simulink model "AEB_Stateflow"  (R2025b)
settings: Solver=ode3  StartTime=0.0  StopTime=15.0  FixedStep=0.001  RelTol=1e-3
values from neighbouring files (symbols this model uses):
  CTRL_DT = 0.01    [AEB_Stateflow_build.m]
  D_BRAKE_L1 = 20.0    (= 20)    [AEB_Stateflow_build.m]
  D_BRAKE_L2 = 10.0    (= 10)    [AEB_Stateflow_build.m]
  D_BRAKE_L3 = 5.0    (= 5)    [AEB_Stateflow_build.m]
  DECEL_BRAKE_L1 = 2.0    (= 2)    [AEB_Stateflow_build.m]
  DECEL_BRAKE_L2 = 4.0    (= 4)    [AEB_Stateflow_build.m]
  DECEL_BRAKE_L3 = 6.0    (= 6)    [AEB_Stateflow_build.m]
  HYSTERESIS_TIME = 0.2    [AEB_Stateflow_build.m]
  POST_BRAKE_TIME = 2.0    (= 2)    [AEB_Stateflow_build.m]
  STEERING_DEG = 5.0    (= 5)    [AEB_Stateflow_build.m]
  TTC_BRAKE_L1 = 3.0    (= 3)    [AEB_Stateflow_build.m]
  TTC_BRAKE_L2 = 2.2    [AEB_Stateflow_build.m]
  TTC_BRAKE_L3 = 1.8    [AEB_Stateflow_build.m]
  TTC_WARNING = 4.0    (= 4)    [AEB_Stateflow_build.m]
  V_EGO_MAX = 16.67    [AEB_Stateflow_build.m]
  V_EGO_MIN = 1.39    [AEB_Stateflow_build.m]
  WARNING_MIN_TIME = 0.8    [AEB_Stateflow_build.m]
settings Model: Creator=rfagu  LastModifiedBy=rfagu

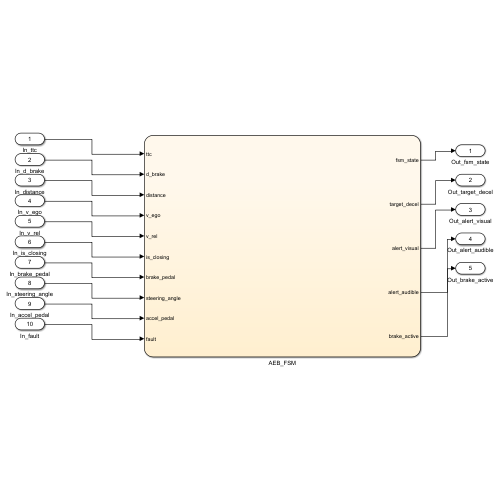
[thumbnail: Simulink's stored preview of the top-level diagram]
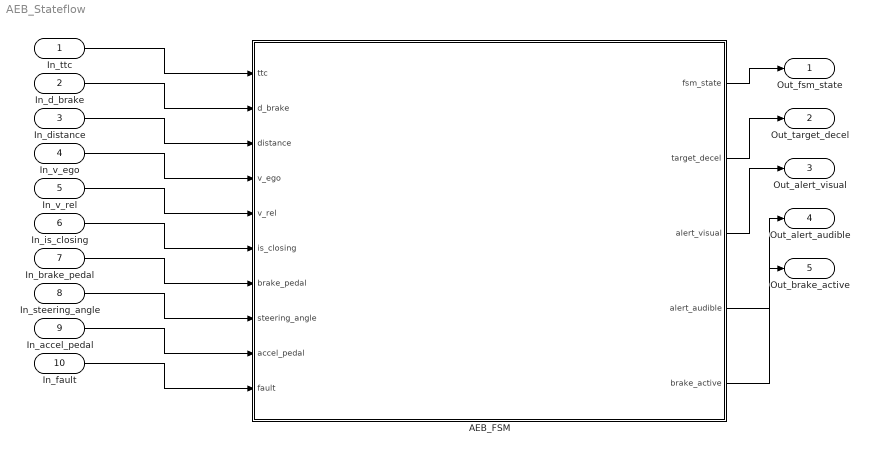
== system AEB_Stateflow ==
  In_ttc : Inport
  In_d_brake : Inport  Port=2
  In_distance : Inport  Port=3
  In_v_ego : Inport  Port=4
  In_v_rel : Inport  Port=5
  In_is_closing : Inport  Port=6
  In_brake_pedal : Inport  Port=7
  In_steering_angle : Inport  Port=8
  In_accel_pedal : Inport  Port=9
  In_fault : Inport  Port=10
  AEB_FSM : Stateflow chart  TreatAsAtomicUnit=on
  Out_fsm_state : Outport
  Out_target_decel : Outport  Port=2
  Out_alert_visual : Outport  Port=3
  Out_alert_audible : Outport  Port=4
  Out_brake_active : Outport  Port=5
  wires:
  In_ttc/1 -> AEB_FSM/1(ttc)
  In_d_brake/1 -> AEB_FSM/2(d_brake)
  In_distance/1 -> AEB_FSM/3(distance)
  In_v_ego/1 -> AEB_FSM/4(v_ego)
  In_v_rel/1 -> AEB_FSM/5(v_rel)
  In_is_closing/1 -> AEB_FSM/6(is_closing)
  In_brake_pedal/1 -> AEB_FSM/7(brake_pedal)
  In_steering_angle/1 -> AEB_FSM/8(steering_angle)
  In_accel_pedal/1 -> AEB_FSM/9(accel_pedal)
  In_fault/1 -> AEB_FSM/10(fault)
  AEB_FSM/1(fsm_state) -> Out_fsm_state/1
  AEB_FSM/2(target_decel) -> Out_target_decel/1
  AEB_FSM/3(alert_visual) -> Out_alert_visual/1
  AEB_FSM/4(alert_audible) -> Out_alert_audible/1
  AEB_FSM/5(brake_active) -> Out_brake_active/1

== stateflow chart AEB_Stateflow/AEB_FSM ==
  settings: updateMethod=DISCRETE  sampleTime=0.01
  state OFF
    entry:
    fsm_state = 0;
    target_decel = 0.0;
    alert_visual = false;
    alert_audible = false;
    brake_active = false;
    debounce_timer = 0.0;
    warning_entry_time = 0.0;
    post_brake_timer = 0.0;
    desired_state = 0.0;
  state STANDBY
    entry:
    fsm_state = 1;
    target_decel = 0.0;
    alert_visual = false;
    alert_audible = false;
    brake_active = false;
    debounce_timer = 0.0;
    warning_entry_time = 0.0;
    post_brake_timer = 0.0;
    desired_state = 1.0;
  state WARNING
    entry:
    fsm_state = 2;
    target_decel = 0.0;
    alert_visual = true;
    alert_audible = true;
    brake_active = false;
    debounce_timer = 0.0;
    warning_entry_time = 0.0;
    desired_state = 2.0;
    during:
    warning_entry_time = warning_entry_time + CTRL_DT;
    if ~is_closing
    desired_state = 1;
    elseif ttc <= TTC_BRAKE_L3 || (d_brake >= distance)
    desired_state = 5;
    elseif ttc <= TTC_BRAKE_L2
    desired_state = 4;
    elseif ttc <= TTC_BRAKE_L1
    desired_state = 3;
    elseif ttc <= TTC_WARNING
    desired_state = 2;
    else
    desired_state = 1;
    end
    %% Distance floor (prevents TTC-based de-escalation when close)
    if is_closing
    if distance <= D_BRAKE_L3 && desired_state < 5
    desired_state = 5;
    elseif distance <= D_BRAKE_L2 && desired_state < 4
    desired_state = 4;
    elseif distance <= D_BRAKE_L1 && desired_state < 3
    desired_state = 3;
    end
    end
    if desired_state < 2
    debounce_timer = debounce_timer + CTRL_DT;
    else
    debounce_timer = 0.0;
    end
  state BRAKE_L1
    entry:
    fsm_state = 3;
    target_decel = DECEL_BRAKE_L1;
    alert_visual = true;
    alert_audible = true;
    brake_active = true;
    debounce_timer = 0.0;
    desired_state = 3.0;
    during:
    if ~is_closing
    desired_state = 1;
    elseif ttc <= TTC_BRAKE_L3 || (d_brake >= distance)
    desired_state = 5;
    elseif ttc <= TTC_BRAKE_L2
    desired_state = 4;
    elseif ttc <= TTC_BRAKE_L1
    desired_state = 3;
    elseif ttc <= TTC_WARNING
    desired_state = 2;
    else
    desired_state = 1;
    end
    %% Distance floor (prevents TTC-based de-escalation when close)
    if is_closing
    if distance <= D_BRAKE_L3 && desired_state < 5
    desired_state = 5;
    elseif distance <= D_BRAKE_L2 && desired_state < 4
    desired_state = 4;
    elseif distance <= D_BRAKE_L1 && desired_state < 3
    desired_state = 3;
    end
    end
    if desired_state < 3
    debounce_timer = debounce_timer + CTRL_DT;
    else
    debounce_timer = 0.0;
    end
  state BRAKE_L2
    entry:
    fsm_state = 4;
    target_decel = DECEL_BRAKE_L2;
    alert_visual = true;
    alert_audible = true;
    brake_active = true;
    debounce_timer = 0.0;
    desired_state = 4.0;
    during:
    if ~is_closing
    desired_state = 1;
    elseif ttc <= TTC_BRAKE_L3 || (d_brake >= distance)
    desired_state = 5;
    elseif ttc <= TTC_BRAKE_L2
    desired_state = 4;
    elseif ttc <= TTC_BRAKE_L1
    desired_state = 3;
    elseif ttc <= TTC_WARNING
    desired_state = 2;
    else
    desired_state = 1;
    end
    %% Distance floor (prevents TTC-based de-escalation when close)
    if is_closing
    if distance <= D_BRAKE_L3 && desired_state < 5
    desired_state = 5;
    elseif distance <= D_BRAKE_L2 && desired_state < 4
    desired_state = 4;
    elseif distance <= D_BRAKE_L1 && desired_state < 3
    desired_state = 3;
    end
    end
    if desired_state < 4
    debounce_timer = debounce_timer + CTRL_DT;
    else
    debounce_timer = 0.0;
    end
  state BRAKE_L3
    entry:
    fsm_state = 5;
    target_decel = DECEL_BRAKE_L3;
    alert_visual = true;
    alert_audible = true;
    brake_active = true;
    debounce_timer = 0.0;
    desired_state = 5.0;
    during:
    if ~is_closing
    desired_state = 1;
    elseif ttc <= TTC_BRAKE_L3 || (d_brake >= distance)
    desired_state = 5;
    elseif ttc <= TTC_BRAKE_L2
    desired_state = 4;
    elseif ttc <= TTC_BRAKE_L1
    desired_state = 3;
    elseif ttc <= TTC_WARNING
    desired_state = 2;
    else
    desired_state = 1;
    end
    %% Distance floor (prevents TTC-based de-escalation when close)
    if is_closing
    if distance <= D_BRAKE_L3 && desired_state < 5
    desired_state = 5;
    elseif distance <= D_BRAKE_L2 && desired_state < 4
    desired_state = 4;
    elseif distance <= D_BRAKE_L1 && desired_state < 3
    desired_state = 3;
    end
    end
    if desired_state < 5
    debounce_timer = debounce_timer + CTRL_DT;
    else
    debounce_timer = 0.0;
    end
  state POST_BRAKE
    entry:
    fsm_state = 6;
    target_decel = DECEL_BRAKE_L3;
    alert_visual = true;
    alert_audible = false;
    brake_active = true;
    post_brake_timer = 0.0;
    debounce_timer = 0.0;
    desired_state = 6.0;
    during:
    post_brake_timer = post_brake_timer + CTRL_DT;
  WARNING -> OFF [order 1] : [fault]
  BRAKE_L3 -> OFF [order 1] : [fault]
  STANDBY -> OFF [order 1] : [fault]
  BRAKE_L2 -> OFF [order 1] : [fault]
  POST_BRAKE -> OFF [order 1] : [fault]
  WARNING -> STANDBY [order 2] : [~fault && (v_ego < V_EGO_MIN || v_ego > V_EGO_MAX)]
  WARNING -> STANDBY [order 3] : [~fault && (brake_pedal || abs(steering_angle) > STEERING_DEG)]
  WARNING -> STANDBY [order 7] : [~fault && v_ego >= V_EGO_MIN && v_ego <= V_EGO_MAX && desired_state <= 1 && debounce_timer >= HYSTERESIS_TIME]
  (default) -> STANDBY
  BRAKE_L1 -> OFF [order 1] : [fault]
  WARNING -> BRAKE_L1 [order 6] : [~fault && v_ego >= V_EGO_MIN && v_ego <= V_EGO_MAX && desired_state == 3 && warning_entry_time >= WARNING_MIN_TIME]
  WARNING -> BRAKE_L2 [order 5] : [~fault && v_ego >= V_EGO_MIN && v_ego <= V_EGO_MAX && desired_state == 4 && warning_entry_time >= WARNING_MIN_TIME]
  BRAKE_L1 -> STANDBY [order 2] : [~fault && (v_ego < V_EGO_MIN || v_ego > V_EGO_MAX)]
  BRAKE_L1 -> STANDBY [order 3] : [~fault && (brake_pedal || abs(steering_angle) > STEERING_DEG)]
  POST_BRAKE -> STANDBY [order 2] : [~fault && accel_pedal]
  POST_BRAKE -> STANDBY [order 3] : [~fault && post_brake_timer >= POST_BRAKE_TIME]
  BRAKE_L2 -> STANDBY [order 2] : [~fault && (v_ego < V_EGO_MIN || v_ego > V_EGO_MAX)]
  BRAKE_L2 -> STANDBY [order 3] : [~fault && (brake_pedal || abs(steering_angle) > STEERING_DEG)]
  OFF -> STANDBY : [~fault]
  BRAKE_L3 -> STANDBY [order 2] : [~fault && (v_ego < V_EGO_MIN || v_ego > V_EGO_MAX)]
  BRAKE_L3 -> STANDBY [order 3] : [~fault && (brake_pedal || abs(steering_angle) > STEERING_DEG)]
  BRAKE_L1 -> WARNING [order 7] : [~fault && v_ego >= V_EGO_MIN && v_ego <= V_EGO_MAX && v_ego > 0.01 && desired_state < 3 && debounce_timer >= HYSTERESIS_TIME]
  STANDBY -> WARNING [order 2] : [~fault && v_ego >= V_EGO_MIN && v_ego <= V_EGO_MAX && is_closing && (ttc <= TTC_WARNING || d_brake >= distance || distance <= D_BRAKE_L1)]
  BRAKE_L3 -> BRAKE_L1 [order 6] : [~fault && v_ego >= V_EGO_MIN && v_ego <= V_EGO_MAX && v_ego > 0.01 && desired_state == 3 && debounce_timer >= HYSTERESIS_TIME]
  BRAKE_L3 -> BRAKE_L2 [order 5] : [~fault && v_ego >= V_EGO_MIN && v_ego <= V_EGO_MAX && v_ego > 0.01 && desired_state == 4 && debounce_timer >= HYSTERESIS_TIME]
  WARNING -> BRAKE_L3 [order 4] : [~fault && v_ego >= V_EGO_MIN && v_ego <= V_EGO_MAX && desired_state == 5 && warning_entry_time >= WARNING_MIN_TIME]
  BRAKE_L2 -> BRAKE_L1 [order 6] : [~fault && v_ego >= V_EGO_MIN && v_ego <= V_EGO_MAX && v_ego > 0.01 && desired_state < 4 && debounce_timer >= HYSTERESIS_TIME]
  BRAKE_L1 -> BRAKE_L2 [order 6] : [~fault && v_ego >= V_EGO_MIN && v_ego <= V_EGO_MAX && v_ego > 0.01 && desired_state == 4]
  BRAKE_L3 -> POST_BRAKE [order 4] : [~fault && v_ego >= V_EGO_MIN && v_ego <= V_EGO_MAX && v_ego <= 0.01]
  BRAKE_L3 -> POST_BRAKE [order 7] : [~fault && v_ego >= V_EGO_MIN && v_ego <= V_EGO_MAX && v_ego > 0.01 && desired_state <= 2 && debounce_timer >= HYSTERESIS_TIME]
  BRAKE_L1 -> BRAKE_L3 [order 5] : [~fault && v_ego >= V_EGO_MIN && v_ego <= V_EGO_MAX && v_ego > 0.01 && desired_state == 5]
  BRAKE_L2 -> BRAKE_L3 [order 5] : [~fault && v_ego >= V_EGO_MIN && v_ego <= V_EGO_MAX && v_ego > 0.01 && desired_state == 5]
  BRAKE_L1 -> POST_BRAKE [order 4] : [~fault && v_ego >= V_EGO_MIN && v_ego <= V_EGO_MAX && v_ego <= 0.01]
  BRAKE_L2 -> POST_BRAKE [order 4] : [~fault && v_ego >= V_EGO_MIN && v_ego <= V_EGO_MAX && v_ego <= 0.01]
  data: ttc input double; d_brake input double; distance input double; v_ego input double; v_rel input double; is_closing input boolean; brake_pedal input boolean; steering_angle input double; accel_pedal input boolean; fault input boolean; fsm_state output double =0; target_decel output double =0; alert_visual output boolean =0; alert_audible output boolean =0; brake_active output boolean =0; warning_entry_time local double =0.0; debounce_timer local double =0.0; post_brake_timer local double =0.0; desired_state local double =1.0; TTC_WARNING parameter double; TTC_BRAKE_L1 parameter double; TTC_BRAKE_L2 parameter double; TTC_BRAKE_L3 parameter double; DECEL_BRAKE_L1 parameter double; DECEL_BRAKE_L2 parameter double; DECEL_BRAKE_L3 parameter double; V_EGO_MIN parameter double; V_EGO_MAX parameter double; HYSTERESIS_TIME parameter double; STEERING_DEG parameter double; POST_BRAKE_TIME parameter double; WARNING_MIN_TIME parameter double; CTRL_DT parameter double; D_BRAKE_L1 parameter double; D_BRAKE_L2 parameter double; D_BRAKE_L3 parameter double
